simulink model "A11_1_sim"  (R2024a)
settings: Solver=ode4  StartTime=0.0  StopTime=14  RelTol=1e-3
values from neighbouring files (symbols this model uses):
  A = [0, 1, 0; 0, 0, 1; 0, -4, -5]    [PA11_1.m]
  B = [0; 0; 1]    [PA11_1.m]
  C = [4, 0, 0]    [PA11_1.m]
  Ki = K(1)    [PA11_1.m]
  Kr = [0, K(2), K(3)]    [PA11_1.m]
  theta_ref = 4*2*pi    (= 25.1327412287)    [PA11_1.m]
settings Model: Creator=caugu  LastModifiedBy=caugu

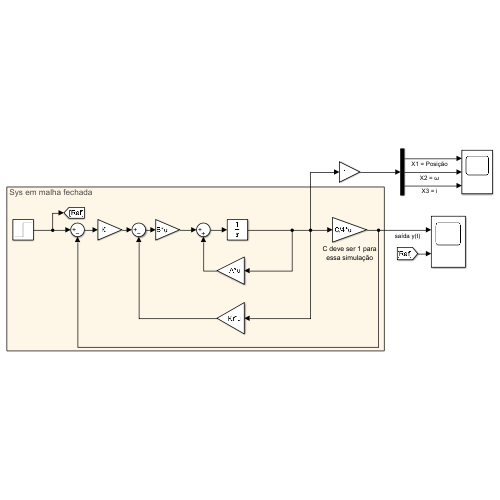
[thumbnail: Simulink's stored preview of the top-level diagram]
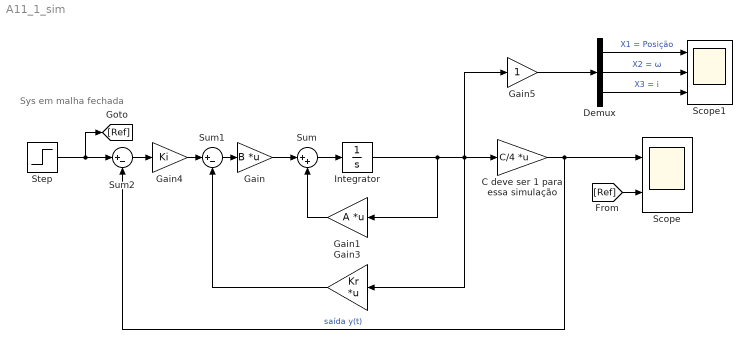
== system A11_1_sim ==
  note: Sys em malha fechada
  C deve ser 1 para essa simulação : Gain  Gain=C/4  Multiplication=Matrix(K*u)
  Demux : Demux  Outputs=3
  Gain : Gain  Gain=B  Multiplication=Matrix(K*u)
  Gain1 : Gain  Gain=A  Multiplication=Matrix(K*u)
  Gain3 : Gain  Gain=Kr  Multiplication=Matrix(K*u)
  Gain4 : Gain  Gain=Ki
  Gain5 : Gain
  Integrator : Integrator
  Scope : Scope  NumInputPorts=2
  Scope1 : Scope  NumInputPorts=3
  Step : Step  After=theta_ref  SampleTime=0
  Sum : Sum  Inputs=|++
  Sum1 : Sum  Inputs=|+-
  Sum2 : Sum  Inputs=|+-
  wires:
  Gain3/1 -> Sum1/2
  Gain1/1 -> Sum/2
  Demux/2 -> Scope1/2  "X2 = ω"
  Demux/1 -> Scope1/1  "X1 = Posição"
  Demux/3 -> Scope1/3  "X3 = i"
  Gain5/1 -> Demux/1
  Sum1/1 -> Gain/1
  Sum2/1 -> Gain4/1
  Gain4/1 -> Sum1/1
  C deve ser 1 para essa simulação/1 -> Sum2/2, Scope/1  "saída y(t)"
  Sum/1 -> Integrator/1
  Gain/1 -> Sum/1
  Integrator/1 -> Gain5/1, Gain3/1, C deve ser 1 para essa simulação/1, Gain1/1
  Step/1 -> [Ref], Sum2/1
  [Ref] -> Scope/2
